simulink model "model_AllInOne1 (1)"  (R2013a)
settings: Solver=ode45  StartTime=0.0  StopTime=400  RelTol=1e-3
undefined symbols (not defined in the file or in its folder): generateDummyBeams, m, s
libraries: test_library x15, aerolib6dofsys x2, aerolibtransform2 x1, aerolibutil x1, aerolibconvert2 x1, falter_library x1, vrlib x1
(part 2 of 2)

== system model_AllInOne1 (1)/Physical Model/6DoF (Euler Angles), incl. gravity and ground detection/pass through ==
  In1 : Inport
  Action Port : ActionPort  ActionType=then
  Fn = zero : Outport
  wires:
  In1/1 -> Fn = zero/1

== system model_AllInOne1 (1)/Physical Model/6DoF (Euler Angles), incl. gravity and ground detection/transform to Inertial axes  ==
  x y z : Inport
  transform coefficients : Inport  Port=2
  Product : Product  Multiplication=Matrix(*)  SaturateOnIntegerOverflow=on  InputSameDT=on  OutDataTypeStr=Inherit: Same as first input
  Reshape1 : Reshape  OutputDimensionality=Column vector (2-D)
  Reshape2 : Reshape
  Ve : Outport
  wires:
  Reshape2/1 -> Ve/1
  Reshape1/1 -> Product/2
  x y z/1 -> Reshape1/1
  transform coefficients/1 -> Product/1
  Product/1 -> Reshape2/1

== system model_AllInOne1 (1)/Physical Model/6DoF (Euler Angles), incl. gravity and ground detection/transform to Inertial axes 1 ==
  x y z : Inport
  transform coefficients : Inport  Port=2
  Product : Product  Multiplication=Matrix(*)  SaturateOnIntegerOverflow=on  InputSameDT=on  OutDataTypeStr=Inherit: Same as first input
  Reshape1 : Reshape  OutputDimensionality=Column vector (2-D)
  Reshape2 : Reshape
  Ve : Outport
  wires:
  Reshape2/1 -> Ve/1
  Reshape1/1 -> Product/2
  x y z/1 -> Reshape1/1
  transform coefficients/1 -> Product/1
  Product/1 -> Reshape2/1

== system model_AllInOne1 (1)/Physical Model/6DoF (Euler Angles), incl. gravity and ground detection/gte zero only/pass through A1 ==
  A_in : Inport
  Action Port : ActionPort  ActionType=then
  A_out : Outport
  wires:
  A_in/1 -> A_out/1

== system model_AllInOne1 (1)/Physical Model/6DoF (Euler Angles), incl. gravity and ground detection/gte zero only/zeroFn ==
  In1 : Inport
  Action Port : ActionPort  ActionType=else
  zero_Fn : Outport
  wires:
  In1/1 -> zero_Fn/1
